simulink model "Teleoperation_Task_Space"  (R2021b)
settings: Solver=FixedStepAuto  StartTime=0.0  StopTime=20  FixedStep=Ts  RelTol=1e-3
values from neighbouring files (symbols this model uses):
  alphas_m = 75.0 * ones(1,dh.dof_task)    [setup_teleop.m]
  alphas_s = alphas_m    [setup_teleop.m]
  B_m = diag(ones(1,dh.dof_task)) * 100    [setup_teleop.m]
  B_s = diag(ones(1,dh.dof_task)) * 15    [setup_teleop.m]
  Fh_A = [1 4*wc 6*wc^2 4*wc^3 wc^4]    [setup_teleop.m]
  Fh_B = [0 0 0 0 wc^4]    [setup_teleop.m]
  gravity = [0 0 9.81]'    [setup_robot.m]
  K_g = eye(dh.dof_task) * k_g    [setup_teleop.m]
  K_m = diag(ones(1,dh.dof_task)) * 0    [setup_teleop.m]
  K_s = diag(ones(1,dh.dof_task)) * 75    [setup_teleop.m]
  KD_e = zeros(dh.dof_task); KD_e(1,1) = 10    [setup_teleop.m]
  KD_h = eye(dh.dof_task) * 50.0    [setup_teleop.m]
  KE_e = zeros(dh.dof_task); KE_e(1,1) = 100    [setup_teleop.m]
  KP_h = eye(dh.dof_task) * 350.0    [setup_teleop.m]
  lambdas_m = 4.0 * ones(1,dh.dof_task)    [setup_teleop.m]
  lambdas_s = lambdas_m    [setup_teleop.m]
  M_m = diag(ones(1,dh.dof_task)) * 1    [setup_teleop.m]
  M_s = diag(ones(1,dh.dof_task)) * 1    [setup_teleop.m]
  T_m2s = 25 / 1000 / Ts    (= 25)    [setup_teleop.m]
  T_s2m = 25 / 1000 / Ts    (= 25)    [setup_teleop.m]
  td = [            0            1                          10            18 ]    [setup_teleop.m]
  Xe = conf.init.x0    [setup_teleop.m]
  zdq_A = [1 4*wc 6*wc^2 4*wc^3 wc^4]    [setup_teleop.m]
  zdq_B = [0 0 0 0 wc^4]    [setup_teleop.m]
undefined symbols (not defined in the file or in its folder): conf_m, conf_s, dh, Fm_A, Fm_B, Fs_A, Fs_B, x0
libraries: vrlib x2, robotcorelib x1, simulink x1
(part 2 of 2)

== system Teleoperation_Task_Space/Sensors/Master Sensors/External Forces ==
  F_in : Inport
  F^_in : Inport  Port=2
  Fd_in : Inport  Port=3
  F : Demux  Outputs=dh.dof
  F^ : Demux  Outputs=dh.dof
  Fd : Demux  Outputs=dh.dof
  Master Fh : Scope  NumInputPorts=6
  Mux{,1..5} (6 alike) : Mux  Inputs=3
  wires:
  F_in/1 -> F/1
  F^_in/1 -> F^/1
  Fd/6 -> Mux5/3
  F/3 -> Mux2/1
  Fd/3 -> Mux2/3
  Mux5/1 -> Master Fh/6
  F^/3 -> Mux2/2
  Fd/1 -> Mux/3
  F^/1 -> Mux/2
  Mux/1 -> Master Fh/1
  F^/2 -> Mux1/2
  Mux1/1 -> Master Fh/2
  Mux3/1 -> Master Fh/4
  F^/6 -> Mux5/2
  F/2 -> Mux1/1
  F/6 -> Mux5/1
  Fd/4 -> Mux3/3
  F/1 -> Mux/1
  Fd/5 -> Mux4/3
  F/4 -> Mux3/1
  Mux2/1 -> Master Fh/3
  F/5 -> Mux4/1
  F^/4 -> Mux3/2
  F^/5 -> Mux4/2
  Fd/2 -> Mux1/3
  Mux4/1 -> Master Fh/5
  Fd_in/1 -> Fd/1

== system Teleoperation_Task_Space/Sensors/Master Sensors/Pose ==
  X_in : Inport
  X^_in : Inport  Port=2
  Xd_in : Inport  Port=3
  Master Pose : Scope  NumInputPorts=6
  Mux{,1..5} (6 alike) : Mux  Inputs=3
  X : Demux  Outputs=dh.dof
  X^ : Demux  Outputs=dh.dof
  Xd : Demux  Outputs=dh.dof
  wires:
  X_in/1 -> X/1
  X/1 -> Mux/1
  X/2 -> Mux1/1
  Mux/1 -> Master Pose/1
  Mux1/1 -> Master Pose/2
  X^/2 -> Mux1/2
  X^_in/1 -> X^/1
  X^/1 -> Mux/2
  Xd/1 -> Mux/3
  Xd/2 -> Mux1/3
  Xd_in/1 -> Xd/1
  Mux2/1 -> Master Pose/3
  Mux3/1 -> Master Pose/4
  Mux4/1 -> Master Pose/5
  Mux5/1 -> Master Pose/6
  X/3 -> Mux2/1
  X/4 -> Mux3/1
  X/5 -> Mux4/1
  X/6 -> Mux5/1
  X^/3 -> Mux2/2
  X^/4 -> Mux3/2
  X^/5 -> Mux4/2
  X^/6 -> Mux5/2
  Xd/3 -> Mux2/3
  Xd/4 -> Mux3/3
  Xd/5 -> Mux4/3
  Xd/6 -> Mux5/3

== system Teleoperation_Task_Space/Sensors/Master Sensors/Speed ==
  dX_in : Inport
  dX^_in : Inport  Port=2
  dXd_in : Inport  Port=3
  Master Speed : Scope  NumInputPorts=6
  Mux{,1..5} (6 alike) : Mux  Inputs=3
  dX : Demux  Outputs=dh.dof
  dX^ : Demux  Outputs=dh.dof
  dXd : Demux  Outputs=dh.dof
  wires:
  dX_in/1 -> dX/1
  dX^_in/1 -> dX^/1
  dXd_in/1 -> dXd/1
  dX^/6 -> Mux5/3
  dX/3 -> Mux2/1
  dX^/3 -> Mux2/3
  Mux5/1 -> Master Speed/6
  dXd/3 -> Mux2/2
  dX^/1 -> Mux/3
  dXd/1 -> Mux/2
  Mux/1 -> Master Speed/1
  dXd/2 -> Mux1/2
  Mux1/1 -> Master Speed/2
  Mux3/1 -> Master Speed/4
  dXd/6 -> Mux5/2
  dX/2 -> Mux1/1
  dX/6 -> Mux5/1
  dX^/4 -> Mux3/3
  dX/1 -> Mux/1
  dX^/5 -> Mux4/3
  dX/4 -> Mux3/1
  Mux2/1 -> Master Speed/3
  dX/5 -> Mux4/1
  dXd/4 -> Mux3/2
  dXd/5 -> Mux4/2
  dX^/2 -> Mux1/3
  Mux4/1 -> Master Speed/5

== system Teleoperation_Task_Space/Sensors/Master Sensors/State ==
  q_in : Inport
  q^_in : Inport  Port=2
  qd_in : Inport  Port=3
  Master State : Scope  NumInputPorts=6
  Mux{,1..5} (6 alike) : Mux  Inputs=3
  q : Demux  Outputs=dh.dof
  q^ : Demux  Outputs=dh.dof
  qd : Demux  Outputs=dh.dof
  wires:
  q_in/1 -> q/1
  qd_in/1 -> qd/1
  q^_in/1 -> q^/1
  qd/6 -> Mux5/3
  q/3 -> Mux2/1
  qd/3 -> Mux2/3
  Mux5/1 -> Master State/6
  q^/3 -> Mux2/2
  qd/1 -> Mux/3
  q^/1 -> Mux/2
  Mux/1 -> Master State/1
  q^/2 -> Mux1/2
  Mux1/1 -> Master State/2
  Mux3/1 -> Master State/4
  q^/6 -> Mux5/2
  q/2 -> Mux1/1
  q/6 -> Mux5/1
  qd/4 -> Mux3/3
  q/1 -> Mux/1
  qd/5 -> Mux4/3
  q/4 -> Mux3/1
  Mux2/1 -> Master State/3
  q/5 -> Mux4/1
  q^/4 -> Mux3/2
  q^/5 -> Mux4/2
  qd/2 -> Mux1/3
  Mux4/1 -> Master State/5

== system Teleoperation_Task_Space/Sensors/Master Sensors/Velocity ==
  dq_in : Inport
  dq^_in : Inport  Port=2
  dqd_in : Inport  Port=3
  Master Velocity : Scope  NumInputPorts=6
  Mux{,1..5} (6 alike) : Mux  Inputs=3
  dq : Demux  Outputs=dh.dof
  dq^ : Demux  Outputs=dh.dof
  dqd : Demux  Outputs=dh.dof
  wires:
  dq_in/1 -> dq/1
  dqd_in/1 -> dqd/1
  dq^_in/1 -> dq^/1
  dqd/6 -> Mux5/3
  dq/3 -> Mux2/1
  dqd/3 -> Mux2/3
  Mux5/1 -> Master Velocity/6
  dq^/3 -> Mux2/2
  dqd/1 -> Mux/3
  dq^/1 -> Mux/2
  Mux/1 -> Master Velocity/1
  dq^/2 -> Mux1/2
  Mux1/1 -> Master Velocity/2
  Mux3/1 -> Master Velocity/4
  dq^/6 -> Mux5/2
  dq/2 -> Mux1/1
  dq/6 -> Mux5/1
  dqd/4 -> Mux3/3
  dq/1 -> Mux/1
  dqd/5 -> Mux4/3
  dq/4 -> Mux3/1
  Mux2/1 -> Master Velocity/3
  dq/5 -> Mux4/1
  dq^/4 -> Mux3/2
  dq^/5 -> Mux4/2
  dqd/2 -> Mux1/3
  Mux4/1 -> Master Velocity/5

== system Teleoperation_Task_Space/Sensors/Slave Sensors/External Forces ==
  F_in : Inport
  F^_in : Inport  Port=2
  Fd_in : Inport  Port=3
  F : Demux  Outputs=dh.dof
  F^ : Demux  Outputs=dh.dof
  Fd : Demux  Outputs=dh.dof
  Mux{,1..5} (6 alike) : Mux  Inputs=3
  Slave Fe : Scope  NumInputPorts=6
  wires:
  F_in/1 -> F/1
  F^_in/1 -> F^/1
  Fd/6 -> Mux5/3
  F/3 -> Mux2/1
  Fd/3 -> Mux2/3
  Mux5/1 -> Slave Fe/6
  F^/3 -> Mux2/2
  Fd/1 -> Mux/3
  F^/1 -> Mux/2
  Mux/1 -> Slave Fe/1
  F^/2 -> Mux1/2
  Mux1/1 -> Slave Fe/2
  Mux3/1 -> Slave Fe/4
  F^/6 -> Mux5/2
  F/2 -> Mux1/1
  F/6 -> Mux5/1
  Fd/4 -> Mux3/3
  F/1 -> Mux/1
  Fd/5 -> Mux4/3
  F/4 -> Mux3/1
  Mux2/1 -> Slave Fe/3
  F/5 -> Mux4/1
  F^/4 -> Mux3/2
  F^/5 -> Mux4/2
  Fd/2 -> Mux1/3
  Mux4/1 -> Slave Fe/5
  Fd_in/1 -> Fd/1

== system Teleoperation_Task_Space/Sensors/Slave Sensors/Pose ==
  X_in : Inport
  X^_in : Inport  Port=2
  Xd_in : Inport  Port=3
  Mux{,1..5} (6 alike) : Mux  Inputs=3
  Slave Pose : Scope  NumInputPorts=6
  X : Demux  Outputs=dh.dof
  X^ : Demux  Outputs=dh.dof
  Xd : Demux  Outputs=dh.dof
  wires:
  X_in/1 -> X/1
  X/1 -> Mux/1
  X/2 -> Mux1/1
  Mux/1 -> Slave Pose/1
  Mux1/1 -> Slave Pose/2
  X^/2 -> Mux1/2
  X^_in/1 -> X^/1
  X^/1 -> Mux/2
  Xd/1 -> Mux/3
  Xd/2 -> Mux1/3
  Xd_in/1 -> Xd/1
  Mux2/1 -> Slave Pose/3
  Mux3/1 -> Slave Pose/4
  Mux4/1 -> Slave Pose/5
  Mux5/1 -> Slave Pose/6
  X/3 -> Mux2/1
  X/4 -> Mux3/1
  X/5 -> Mux4/1
  X/6 -> Mux5/1
  X^/3 -> Mux2/2
  X^/4 -> Mux3/2
  X^/5 -> Mux4/2
  X^/6 -> Mux5/2
  Xd/3 -> Mux2/3
  Xd/4 -> Mux3/3
  Xd/5 -> Mux4/3
  Xd/6 -> Mux5/3

== system Teleoperation_Task_Space/Sensors/Slave Sensors/Speed ==
  dX_in : Inport
  dX^_in : Inport  Port=2
  dXd_in : Inport  Port=3
  Mux{,1..5} (6 alike) : Mux  Inputs=3
  Slave Speed : Scope  NumInputPorts=6
  dX : Demux  Outputs=dh.dof
  dX^ : Demux  Outputs=dh.dof
  dXd : Demux  Outputs=dh.dof
  wires:
  dX_in/1 -> dX/1
  dX^_in/1 -> dX^/1
  dXd_in/1 -> dXd/1
  dX^/6 -> Mux5/3
  dX/3 -> Mux2/1
  dX^/3 -> Mux2/3
  Mux5/1 -> Slave Speed/6
  dXd/3 -> Mux2/2
  dX^/1 -> Mux/3
  dXd/1 -> Mux/2
  Mux/1 -> Slave Speed/1
  dXd/2 -> Mux1/2
  Mux1/1 -> Slave Speed/2
  Mux3/1 -> Slave Speed/4
  dXd/6 -> Mux5/2
  dX/2 -> Mux1/1
  dX/6 -> Mux5/1
  dX^/4 -> Mux3/3
  dX/1 -> Mux/1
  dX^/5 -> Mux4/3
  dX/4 -> Mux3/1
  Mux2/1 -> Slave Speed/3
  dX/5 -> Mux4/1
  dXd/4 -> Mux3/2
  dXd/5 -> Mux4/2
  dX^/2 -> Mux1/3
  Mux4/1 -> Slave Speed/5

== system Teleoperation_Task_Space/Sensors/Slave Sensors/State ==
  q_in : Inport
  q^_in : Inport  Port=2
  qd_in : Inport  Port=3
  Mux{,1..5} (6 alike) : Mux  Inputs=3
  Slave State : Scope  NumInputPorts=6
  q : Demux  Outputs=dh.dof
  q^ : Demux  Outputs=dh.dof
  qd : Demux  Outputs=dh.dof
  wires:
  q_in/1 -> q/1
  qd_in/1 -> qd/1
  q^_in/1 -> q^/1
  qd/6 -> Mux5/3
  q/3 -> Mux2/1
  qd/3 -> Mux2/3
  Mux5/1 -> Slave State/6
  q^/3 -> Mux2/2
  qd/1 -> Mux/3
  q^/1 -> Mux/2
  Mux/1 -> Slave State/1
  q^/2 -> Mux1/2
  Mux1/1 -> Slave State/2
  Mux3/1 -> Slave State/4
  q^/6 -> Mux5/2
  q/2 -> Mux1/1
  q/6 -> Mux5/1
  qd/4 -> Mux3/3
  q/1 -> Mux/1
  qd/5 -> Mux4/3
  q/4 -> Mux3/1
  Mux2/1 -> Slave State/3
  q/5 -> Mux4/1
  q^/4 -> Mux3/2
  q^/5 -> Mux4/2
  qd/2 -> Mux1/3
  Mux4/1 -> Slave State/5

== system Teleoperation_Task_Space/Sensors/Slave Sensors/Velocity ==
  dq_in : Inport
  dq^_in : Inport  Port=2
  dqd_in : Inport  Port=3
  Mux{,1..5} (6 alike) : Mux  Inputs=3
  Slave Velocity : Scope  NumInputPorts=6
  dq : Demux  Outputs=dh.dof
  dq^ : Demux  Outputs=dh.dof
  dqd : Demux  Outputs=dh.dof
  wires:
  dq_in/1 -> dq/1
  dqd_in/1 -> dqd/1
  dq^_in/1 -> dq^/1
  dqd/6 -> Mux5/3
  dq/3 -> Mux2/1
  dqd/3 -> Mux2/3
  Mux5/1 -> Slave Velocity/6
  dq^/3 -> Mux2/2
  dqd/1 -> Mux/3
  dq^/1 -> Mux/2
  Mux/1 -> Slave Velocity/1
  dq^/2 -> Mux1/2
  Mux1/1 -> Slave Velocity/2
  Mux3/1 -> Slave Velocity/4
  dq^/6 -> Mux5/2
  dq/2 -> Mux1/1
  dq/6 -> Mux5/1
  dqd/4 -> Mux3/3
  dq/1 -> Mux/1
  dqd/5 -> Mux4/3
  dq/4 -> Mux3/1
  Mux2/1 -> Slave Velocity/3
  dq/5 -> Mux4/1
  dq^/4 -> Mux3/2
  dq^/5 -> Mux4/2
  dqd/2 -> Mux1/3
  Mux4/1 -> Slave Velocity/5

== system Teleoperation_Task_Space/Slave Observer and Force Estimator/Sliding Mode Control/Subsystem1 ==
  s : Inport
  Abs : Abs
  Constant : Constant  Value=10e-5
  Constant1 : Constant  Value=ones(1,dh.dof_task)
  Constant2 : Constant
  Divide : Product  Inputs=*/
  Product : Product
  Product1 : Product
  Relational Operator : RelationalOperator  Operator=>  OutDataTypeStr=boolean  RndMeth=Simplest
  Sign : Signum
  Sum : Sum  Inputs=+-|
  Sum1 : Sum  Inputs=+|+
  sat_x : Outport
  wires:
  Divide/1 -> Product1/2, Sign/1, Abs/1
  s/1 -> Divide/1
  Constant/1 -> Divide/2
  Abs/1 -> Relational Operator/1
  Sum1/1 -> sat_x/1
  Sign/1 -> Product/1
  Constant1/1 -> Relational Operator/2
  Relational Operator/1 -> Sum/2, Product/2
  Constant2/1 -> Sum/1
  Sum/1 -> Product1/1
  Product/1 -> Sum1/1
  Product1/1 -> Sum1/2

== matlab function Teleoperation_Task_Space/Master Robot/Injectable Robot Model (Joint Space)/MATLAB Function1 ==
  data: X output; q input; dh parameter
function X = K(q, dh)
    X = K_rne(dh, q);
end

== matlab function Teleoperation_Task_Space/Master Robot/Injectable Robot Model (Joint Space)/MATLAB Function2 ==
  data: q input; uA input; u output; dh parameter
function u = JAT(q,uA, dh)
    u = JA_rne(dh,q)' * uA;
end

== matlab function Teleoperation_Task_Space/Master Robot/Injectable Robot Model (Joint Space)/MATLAB Function3 ==
  data: dh parameter; dX output; q input; dq input
function dX = JA(dh, q, dq)
    dX = JA_rne(dh, q)*dq;
end

== matlab function Teleoperation_Task_Space/Master Controller/Master Controller ==
  data: dh parameter; qm input size=dh.dof; dqm input size=dh.dof; Xm input size=dh.dof_task; Fm output size=dh.dof_task; dXm input size=dh.dof_task; Fh input size=dh.dof_task; Fe_d input size=dh.dof_task; gravity parameter size=3; M_m parameter size=[dh.dof_task,dh.dof_task]; B_m parameter size=[dh.dof_task,dh.dof_task]; K_m parameter size=[dh.dof_task,dh.dof_task]
function Fm = Cm(dh,qm,dqm, Xm,dXm, Fh,Fe_d,gravity, M_m,B_m,K_m)
    
    BA = BA_rne(dh, qm);
    CAdX = CAdX_rne(dh, qm, dqm);  % we can use CAdX instead of CA*dX since here dq and dX have the same meaning
    GA = GA_rne(dh, qm, gravity);

    % inner impedance controller
    vm = M_m \ (-B_m*dXm - K_m*Xm + Fh - Fe_d);
    % outer decoupling/linearization controller
    Fm = BA*vm + CAdX + GA - Fh;
end

== matlab function Teleoperation_Task_Space/Master Robot/Injectable Robot Model (Joint Space)/MATLAB Function4 ==
  data: q input size=dh.dof; inject_ddq output size=dh.dof; inject_ddX input size=dh.dof_task; dh parameter
function inject_ddq = get_inject_ddq(q, inject_ddX, dh)
    JA = JA_rne(dh, q);
    inject_ddq = pinv(JA) * inject_ddX;
end

== matlab function Teleoperation_Task_Space/Master Robot/Injectable Robot Model (Joint Space)/MATLAB Function5 ==
  data: q input size=dh.dof; inject_dq output size=dh.dof; inject_dX input size=dh.dof_task; dh parameter
function inject_dq = get_inject_dq(q, inject_dX, dh)
    JA = JA_rne(dh, q);
    inject_dq = pinv(JA) * inject_dX;
end

== matlab function Teleoperation_Task_Space/Master Observer and Force Estimator/Injectable Robot Model (Joint Space)/MATLAB Function ==
  data ddq_ settings: updateMethod=SF_CONTINUOUS_TIME_DATA
  data dq_ settings: updateMethod=SF_CONTINUOUS_TIME_DATA
  data dq settings: updateMethod=SF_CONTINUOUS_TIME_DATA
  data q settings: updateMethod=SF_CONTINUOUS_TIME_DATA
  data u settings: updateMethod=SF_CONTINUOUS_TIME_DATA
  data: ddq_ output size=dh.dof; dq_ output size=dh.dof; dq input size=dh.dof; q input size=dh.dof; u input size=dh.dof; g input size=3; dh parameter
function [ddq_, dq_]  = RobotSystem(dq, q, u, g, dh)
    
    % compute dynamics
    B = B_rne(dh, q);
    C = C_rne(dh, q, dq);
    G = G_rne(dh, q, g);

    dq_ = dq(1:dh.dof);

    ddq = B \ (u - C*dq - G);
    ddq_ = ddq(1:dh.dof);
end

== matlab function Teleoperation_Task_Space/Master Observer and Force Estimator/Injectable Robot Model (Joint Space)/MATLAB Function1 ==
  data: X output; q input; dh parameter
function X = K(q, dh)
    X = K_rne(dh, q);
end

== matlab function Teleoperation_Task_Space/Slave Robot/Injectable Robot Model (Joint Space)/MATLAB Function1 ==
  data: X output; q input; dh parameter
function X = K(q, dh)
    X = K_rne(dh, q);
end

== matlab function Teleoperation_Task_Space/Master Observer and Force Estimator/Injectable Robot Model (Joint Space)/MATLAB Function2 ==
  data: q input size=dh.dof; uA input size=dh.dof_task; u output size=dh.dof; dh parameter
function u = JAT(q,uA, dh)
    u = JA_rne(dh,q)' * uA;
end

== matlab function Teleoperation_Task_Space/Master Observer and Force Estimator/Injectable Robot Model (Joint Space)/MATLAB Function3 ==
  data: dh parameter; dX output; q input; dq input
function dX = JA(dh, q, dq)
    dX = JA_rne(dh, q)*dq;
end

== matlab function Teleoperation_Task_Space/Master Observer and Force Estimator/Injectable Robot Model (Joint Space)/MATLAB Function4 ==
  data: q input size=dh.dof; inject_ddq output size=dh.dof; inject_ddX input size=dh.dof_task; dh parameter
function inject_ddq = get_inject_ddq(q, inject_ddX, dh)
    JA = JA_rne(dh, q);
    inject_ddq = pinv(JA) * inject_ddX;
end

== matlab function Teleoperation_Task_Space/Master Observer and Force Estimator/MATLAB Function1 ==
  data: Fh output; q input; zm2eq input; dh parameter
function Fh = BA_zm(q, zm2eq, dh)
     BA = BA_rne(dh, q);
     Fh = BA * zm2eq;
end

== matlab function Teleoperation_Task_Space/Slave Robot/Injectable Robot Model (Joint Space)/MATLAB Function2 ==
  data: q input; uA input; u output; dh parameter
function u = JAT(q,uA, dh)
    u = JA_rne(dh,q)' * uA;
end

== matlab function Teleoperation_Task_Space/Slave Robot/Injectable Robot Model (Joint Space)/MATLAB Function3 ==
  data: dh parameter; dX output; q input; dq input
function dX = JA(dh, q, dq)
    dX = JA_rne(dh, q)*dq;
end

== matlab function Teleoperation_Task_Space/Slave Robot/Injectable Robot Model (Joint Space)/MATLAB Function4 ==
  data: q input size=dh.dof; inject_ddq output size=dh.dof; inject_ddX input size=dh.dof_task; dh parameter
function inject_ddq = get_inject_ddq(q, inject_ddX, dh)
    JA = JA_rne(dh, q);
    inject_ddq = pinv(JA) * inject_ddX;
end

== matlab function Teleoperation_Task_Space/Master Observer and Force Estimator/Injectable Robot Model (Joint Space)/MATLAB Function5 ==
  data: q input size=dh.dof; inject_dq output size=dh.dof; inject_dX input size=dh.dof_task; dh parameter
function inject_dq = get_inject_dq(q, inject_dX, dh)
    JA = JA_rne(dh, q);
    inject_dq = pinv(JA) * inject_dX;
end

== matlab function Teleoperation_Task_Space/Slave Robot/Injectable Robot Model (Joint Space)/MATLAB Function5 ==
  data: q input size=dh.dof; inject_dq output size=dh.dof; inject_dX input size=dh.dof_task; dh parameter
function inject_dq = get_inject_dq(q, inject_dX, dh)
    JA = JA_rne(dh, q);
    inject_dq = pinv(JA) * inject_dX;
end

== matlab function Teleoperation_Task_Space/Slave Observer and Force Estimator/Injectable Robot Model (Joint Space)/MATLAB Function2 ==
  data: q input size=dh.dof; uA input size=dh.dof_task; u output size=dh.dof; dh parameter
function u = JAT(q,uA, dh)
    u = JA_rne(dh,q)' * uA;
end

== matlab function Teleoperation_Task_Space/Slave Observer and Force Estimator/Injectable Robot Model (Joint Space)/MATLAB Function3 ==
  data: dh parameter; dX output; q input; dq input
function dX = JA(dh, q, dq)
    dX = JA_rne(dh, q)*dq;
end

== matlab function Teleoperation_Task_Space/Slave Observer and Force Estimator/Injectable Robot Model (Joint Space)/MATLAB Function4 ==
  data: q input size=dh.dof; inject_ddq output size=dh.dof; inject_ddX input size=dh.dof_task; dh parameter
function inject_ddq = get_inject_ddq(q, inject_ddX, dh)
    JA = JA_rne(dh, q);
    inject_ddq = pinv(JA) * inject_ddX;
end

== matlab function Teleoperation_Task_Space/Slave Robot/Injectable Robot Model (Joint Space)/MATLAB Function ==
  data ddq_ settings: updateMethod=SF_CONTINUOUS_TIME_DATA
  data dq_ settings: updateMethod=SF_CONTINUOUS_TIME_DATA
  data dq settings: updateMethod=SF_CONTINUOUS_TIME_DATA
  data q settings: updateMethod=SF_CONTINUOUS_TIME_DATA
  data u settings: updateMethod=SF_CONTINUOUS_TIME_DATA
  data: ddq_ output size=dh.dof; dq_ output size=dh.dof; dq input size=dh.dof; q input size=dh.dof; u input size=dh.dof; g input size=3; dh parameter
function [ddq_, dq_]  = RobotSystem(dq, q, u, g, dh)
    
    % compute dynamics
    B = B_rne(dh, q);
    C = C_rne(dh, q, dq);
    G = G_rne(dh, q, g);

    dq_ = dq(1:dh.dof);

    ddq = B \ (u - C*dq - G);
    ddq_ = ddq(1:dh.dof);
end

== matlab function Teleoperation_Task_Space/Slave Observer and Force Estimator/Injectable Robot Model (Joint Space)/MATLAB Function5 ==
  data: q input size=dh.dof; inject_dq output size=dh.dof; inject_dX input size=dh.dof_task; dh parameter
function inject_dq = get_inject_dq(q, inject_dX, dh)
    JA = JA_rne(dh, q);
    inject_dq = pinv(JA) * inject_dX;
end

== matlab function Teleoperation_Task_Space/Slave Observer and Force Estimator/MATLAB Function1 ==
  data: Fe output; q input; zs2eq input; dh parameter
function Fe = BA_zm(q, zs2eq, dh)
     BA = BA_rne(dh, q);
     Fe = - BA * zs2eq;
end

== matlab function Teleoperation_Task_Space/Slave Observer and Force Estimator/Injectable Robot Model (Joint Space)/MATLAB Function ==
  data ddq_ settings: updateMethod=SF_CONTINUOUS_TIME_DATA
  data dq_ settings: updateMethod=SF_CONTINUOUS_TIME_DATA
  data dq settings: updateMethod=SF_CONTINUOUS_TIME_DATA
  data q settings: updateMethod=SF_CONTINUOUS_TIME_DATA
  data u settings: updateMethod=SF_CONTINUOUS_TIME_DATA
  data: ddq_ output size=dh.dof; dq_ output size=dh.dof; dq input size=dh.dof; q input size=dh.dof; u input size=dh.dof; g input size=3; dh parameter
function [ddq_, dq_]  = RobotSystem(dq, q, u, g, dh)
    
    % compute dynamics
    B = B_rne(dh, q);
    C = C_rne(dh, q, dq);
    G = G_rne(dh, q, g);

    dq_ = dq(1:dh.dof);

    ddq = B \ (u - C*dq - G);
    ddq_ = ddq(1:dh.dof);
end

== matlab function Teleoperation_Task_Space/Slave Observer and Force Estimator/Injectable Robot Model (Joint Space)/MATLAB Function1 ==
  data: X output; q input; dh parameter
function X = K(q, dh)
    X = K_rne(dh, q);
end

== matlab function Teleoperation_Task_Space/Slave controller/Slave Controller ==
  data: dh parameter; gravity parameter size=3; qs input size=dh.dof; dqs input size=dh.dof; Xs input size=dh.dof_task; Fs output size=dh.dof_task; dXs input size=dh.dof_task; qm input size=dh.dof; Xm input size=dh.dof_task; dXm input size=dh.dof_task; Fh input size=dh.dof_task; Fe input size=dh.dof_task; Fedd input size=dh.dof_task; zs2eq input size=dh.dof_task; zm2eq input size=dh.dof_task; sign_s input size=dh.dof_task; M_m parameter size=[dh.dof_task,dh.dof_task]; B_m parameter size=[dh.dof_task,dh.dof_task]; K_m parameter size=[dh.dof_task,dh.dof_task]; M_s parameter size=[dh.dof_task,dh.dof_task]; B_s parameter size=[dh.dof_task,dh.dof_task]; K_s parameter size=[dh.dof_task,dh.dof_task]; K_g parameter size=[dh.dof_task,dh.dof_task]
function Fs = Cs(dh,gravity, qs,dqs,Xs,dXs, qm,Xm,dXm, Fh,Fe,Fedd, zs2eq,zm2eq,sign_s, M_m,B_m,K_m, M_s,B_s,K_s,K_g)

    MAs = BA_rne(dh, qs);
    if any(~isfinite(MAs))
        MAs = zeros(size(MAs));
    end
    CAdX = CAdX_rne(dh, qs, dqs);
    GAs = GA_rne(dh, qs, gravity);
    hAs = CAdX + GAs;
    % TODO needs the master dh, but in this project we have the same robots
    MAm = BA_rne(dh, qm);
    if any(~isfinite(MAm))
        MAm = zeros(size(MAm));
    end
    
    Fs = -MAs * (M_s\K_s*Xs + M_s\B_s*dXs ...
                - MAs\hAs ...
                + (M_m\K_m - M_s\K_s)*Xm ...
                + (M_m\B_m - M_s\B_s)*dXm ...
                - (inv(M_m) - pinv(MAm))*Fh ...
                + M_m\Fedd + M_s\Fe ...
                + zs2eq + zm2eq + K_g*sign_s);
    Fs = Fs;
end

== matlab function Teleoperation_Task_Space/Master Robot/Injectable Robot Model (Joint Space)/MATLAB Function ==
  data ddq_ settings: updateMethod=SF_CONTINUOUS_TIME_DATA
  data dq_ settings: updateMethod=SF_CONTINUOUS_TIME_DATA
  data dq settings: updateMethod=SF_CONTINUOUS_TIME_DATA
  data q settings: updateMethod=SF_CONTINUOUS_TIME_DATA
  data u settings: updateMethod=SF_CONTINUOUS_TIME_DATA
  data: ddq_ output size=dh.dof; dq_ output size=dh.dof; dq input size=dh.dof; q input size=dh.dof; u input size=dh.dof; g input size=3; dh parameter
function [ddq_, dq_]  = RobotSystem(dq, q, u, g, dh)
    
    % compute dynamics
    B = B_rne(dh, q);
    C = C_rne(dh, q, dq);
    G = G_rne(dh, q, g);

    dq_ = dq(1:dh.dof);

    ddq = B \ (u - C*dq - G);
    ddq_ = ddq(1:dh.dof);
end
